simulink model "SimulinkHW2"  (R2018b)
settings: Solver=VariableStepAuto  StartTime=0.0  StopTime=10.0  RelTol=1e-3
settings Model: Creator=GRosp  LastModifiedBy=GRosp

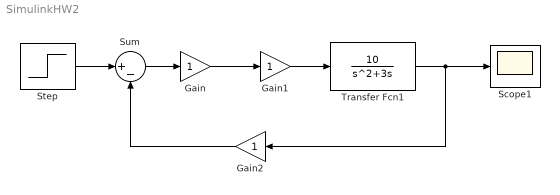
== system SimulinkHW2 ==
  Gain : Gain
  Gain1 : Gain
  Gain2 : Gain
  Scope1 : Scope
  Step : Step  Time=0  SampleTime=0.01
  Sum : Sum  Inputs=|+-
  Transfer Fcn1 : TransferFcn  Numerator=[10]  Denominator=[1 3 0]
  wires:
  Transfer Fcn1/1 -> Gain2/1, Scope1/1
  Step/1 -> Sum/1
  Gain/1 -> Gain1/1
  Sum/1 -> Gain/1
  Gain1/1 -> Transfer Fcn1/1
  Gain2/1 -> Sum/2
